simulink model "HopperRaibert"  (R2025a)
settings: Solver=VariableStepAuto  StartTime=0.0  StopTime=10.0  RelTol=1e-3
libraries: aru_toolbox x2, simulink x1
settings Model: Creator=Gavin  LastModifiedBy=Gavin
settings ExplorerConfigSet: InternalSimMechanicsExplorerSettings="<ExplorerConfiguration><canonicalview>default</canonicalview><TilePanel><TileInfo><Tiles Columns=\"1\" Count=\"1\" Height=\"832\" Rows=\"1\" Width=\"1462\"><Row Weight=\"1\"/><Column Weight=\"1\"/><Tile Height=\"1\" Width=\"1\" X=\"0\" Y=\"0\"/></Tiles></TileInfo><SceneInfo><SceneViewer><IsThisViewStd><IsStandardView>off</IsStandardView><StandardViewName>Front</StandardViewName></IsThisViewStd><BGColor><R>1</R><G>1</G><B>1</B><A>1</A></BGColor><Camera><DoPerspective>on</DoPerspective><Position><X>-0.15165999999999999</X><Y>3.9971199999999998</Y><Z>0.85099999999999998</Z></Position><Center><X>0</X><Y>0</Y><Z>0.10100000000000001</Z></Center><Up><X>0.0069873130929931429</X><Y>-0.18415619748295364</Y><Z>0.98287215464899591</Z></Up><XLim>1.8977346774231529</XLim><YLim>1.8977346774231529</YLim><ViewLimDist>0.01</ViewLimDist></Camera></SceneViewer></SceneInfo></TilePanel><MechEditorPanel><GfxPanelCameraMap><MapElement CameraMLId=\"Camera1\" GfxPanelIndex=\"0\"/></GfxPanelCameraMap><Cameras><Camera><Id>Camera1</Id><Value><Name>FollowBot</Name><NativeCamera><PositionTrackingFeature>Subsystem.Half_Baleka_Simscape_WIP.Planarising_Boom.Center_to_CameraUp.F</PositionTrackingFeature><CenterTrackingFeature>Subsystem.Half_Baleka_Simscape_WIP.Planarising_Boom.Center_to_Camera.B</CenterTrackingFeature><UpVectorTrackingFeature>Subsystem.Half_Baleka_Simscape_WIP.Planarising_Boom.Center_to_Camera.B</UpVectorTrackingFeature><CenterTrackingOrigin>on</CenterTrackingOrigin><UpVectorTrackingDirection>+Y</UpVectorTrackingDirection></NativeCamera></Value></Camera></Cameras><VideoCreator><IncludeTiles>All</IncludeTiles><IncludeTime>on</IncludeTime><IncludeWorldFrame>off</IncludeWorldFrame><PlaybackSpeedRatio>1</PlaybackSpeedRatio><FrameRate>30</FrameRate><FrameSize>auto</FrameSize><VideoFormat>MotionJPEGAVI</VideoFormat></VideoCreator></MechEditorPanel><PlaybackSettings><PlaybackSpeedFactor>1</PlaybackSpeedFactor></PlaybackSettings></ExplorerConfiguration>"

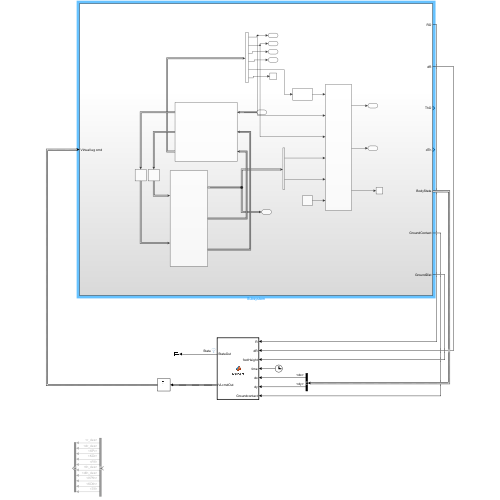
[thumbnail: Simulink's stored preview of the top-level diagram]
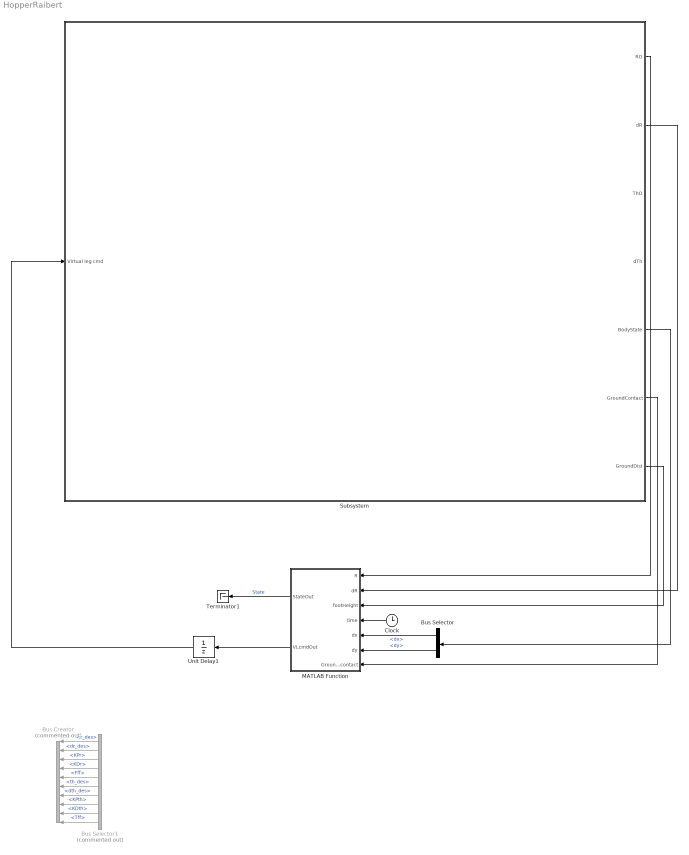
== system HopperRaibert ==
  Bus Creator : BusCreator  Commented=on  Inputs=10  OutDataTypeStr=Bus: VLcmd  NonVirtualBus=on
      settings: InheritFromInputs=off
  Bus Selector : BusSelector  OutputSignals=dx,dy
  Bus Selector1 : BusSelector  Commented=on  OutputSignals=r_des,dr_des,KPr,KDr,Fff,th_des,dth_des,KPth,KDth,Tff
  Clock : Clock
  MATLAB Function : MATLAB Function  TreatAsAtomicUnit=on
  Subsystem : Subsystem
  Terminator1 : Terminator
  Unit Delay1 : UnitDelay  SampleTime=-1  HasFrameUpgradeWarning=on
  wires:
  MATLAB Function/1(StateOut) -> Terminator1/1  "State"
  Subsystem/6(GroundContact) -> MATLAB Function/7(Groundcontact)
  Subsystem/2(dR) -> MATLAB Function/2(dR)
  Clock/1 -> MATLAB Function/4(time)
  Subsystem/1(RO) -> MATLAB Function/1(R)
  Subsystem/7(GroundDist) -> MATLAB Function/3(footHeight)
  Subsystem/5(BodyState) -> Bus Selector/1
  Bus Selector/1 -> MATLAB Function/5(dx)  "<dx>"
  Bus Selector/2 -> MATLAB Function/6(dy)  "<dy>"
  Bus Selector1/8 -> Bus Creator/8  "<KPth>"
  Bus Selector1/2 -> Bus Creator/2  "<dr_des>"
  Bus Selector1/4 -> Bus Creator/4  "<KDr>"
  Bus Selector1/7 -> Bus Creator/7  "<dth_des>"
  Bus Selector1/5 -> Bus Creator/5  "<Fff>"
  Bus Selector1/6 -> Bus Creator/6  "<th_des>"
  Bus Selector1/3 -> Bus Creator/3  "<KPr>"
  Bus Selector1/10 -> Bus Creator/10  "<Tff>"
  Bus Selector1/9 -> Bus Creator/9  "<KDth>"
  Bus Selector1/1 -> Bus Creator/1  "<r_des>"
  MATLAB Function/2(VLcmdOut) -> Unit Delay1/1
  Unit Delay1/1 -> Subsystem/1(Virtual leg cmd)

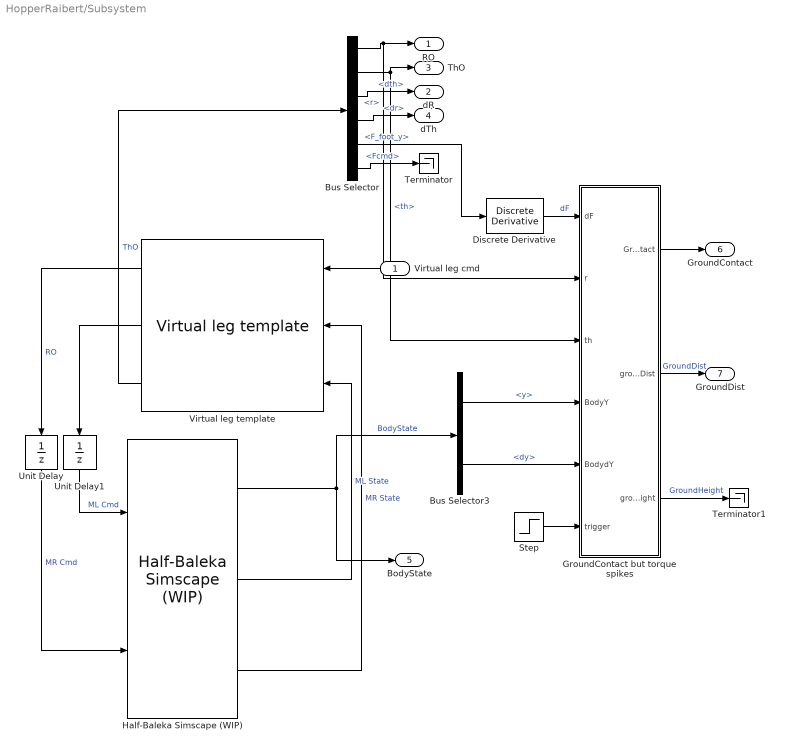
== system HopperRaibert/Subsystem ==
  Virtual leg cmd : Inport  OutDataTypeStr=Bus: VLcmd
  Bus Selector : BusSelector  OutputSignals=r,th,dth,dr,F_foot_y,Fcmd
  Bus Selector3 : BusSelector  OutputSignals=y,dy
  Discrete Derivative : simulink/Discrete/Discrete Derivative  gainval=1.0  ICPrevScaledInput=0.0  OutMin=[]  OutMax=[]  OutDataType=fixdt(1, 16)  OutScaling=2^-10  DoSatur=off
  GroundContact but torque spikes : MATLAB Function  TreatAsAtomicUnit=on
  Half-Baleka Simscape (WIP) : aru_toolbox/Baleka 2.5/Half-Baleka Simscape (WIP)  communication_rate=1000  GravityBool=on  mu_s=1  mu_k=0.9  foot_k=1e5  foot_d=1e4  y_start=0.8  dx_start=2  StartingMode=Zero (set Starting values manually)  LOffset=4.1  ROffset=-0.88  camX=4  camY=0.75
      settings: SourceProductName=ARU Toolbox
  Step : Step  Time=0.005  SampleTime=0
  Terminator : Terminator
  Terminator1 : Terminator
  Unit Delay : UnitDelay  SampleTime=-1  HasFrameUpgradeWarning=on
  Unit Delay1 : UnitDelay  SampleTime=-1  HasFrameUpgradeWarning=on
  Virtual leg template : aru_toolbox/Baleka 2.5/Virtual leg template  SystemSampleTime=-1  VariantActivationTime=update diagram  EmptyChoice=off  PassThrough=off  PassThroughVariantControl=(default)  EmptyChoiceVariantControl=(default)  AllowFlexibleInterface=on  Latency=0  AutoFrameSizeCalculation=off
      settings: SourceProductName=ARU Toolbox
  RO : Outport
  dR : Outport  Port=2
  ThO : Outport  Port=3
  dTh : Outport  Port=4
  BodyState : Outport  Port=5
  GroundContact : Outport  Port=6
  GroundDist : Outport  Port=7
  wires:
  Bus Selector/6 -> Terminator/1  "<Fcmd>"
  Bus Selector/4 -> dTh/1  "<dr>"
  Bus Selector/1 -> GroundContact but torque spikes/2(r), RO/1  "<r>"
  Unit Delay1/1 -> Half-Baleka Simscape (WIP)/1  "ML Cmd"
  Virtual leg cmd/1 -> Virtual leg template/1
  Virtual leg template/3 -> Bus Selector/1  "ThO"
  Half-Baleka Simscape (WIP)/3 -> Virtual leg template/2  "MR State"
  Half-Baleka Simscape (WIP)/2 -> Virtual leg template/3  "ML State"
  Virtual leg template/1 -> Unit Delay/1  "RO"
  Bus Selector/2 -> ThO/1, GroundContact but torque spikes/3(th)  "<th>"
  Unit Delay/1 -> Half-Baleka Simscape (WIP)/2  "MR Cmd"
  Half-Baleka Simscape (WIP)/1 -> BodyState/1, Bus Selector3/1  "BodyState"
  Bus Selector/5 -> Discrete Derivative/1  "<F_foot_y>"
  GroundContact but torque spikes/1(GroundContact) -> GroundContact/1
  Bus Selector/3 -> dR/1  "<dth>"
  Virtual leg template/2 -> Unit Delay1/1
  Bus Selector3/1 -> GroundContact but torque spikes/4(BodyY)  "<y>"
  Bus Selector3/2 -> GroundContact but torque spikes/5(BodydY)  "<dy>"
  GroundContact but torque spikes/3(groundHeight) -> Terminator1/1  "GroundHeight"
  Discrete Derivative/1 -> GroundContact but torque spikes/1(dF)  "dF"
  GroundContact but torque spikes/2(groundDist) -> GroundDist/1  "GroundDist"
  Step/1 -> GroundContact but torque spikes/6(trigger)

== matlab function HopperRaibert/MATLAB Function ==
  settings: updateMethod=DISCRETE  sampleTime=0.001
  data: R input; StateOut output; dR input; footHeight input; time input; dx input; dy input; VLcmdOut output Bus: VLcmd; Groundcontact input
function [StateOut, VLcmdOut]   = Raibert(R, dR,footHeight, time,dx, dy, Groundcontact)
    % Raibert hopping state machine
    persistent state landTime VLcmd x_f_des %dR
    % State variable
    % 0 = SETUP
    % 1 = FLIGHT
    % 2 = COMPRESSION
    % 3 = THRUST
    
    % Params:
    Ts = 0.15;
    Kdx = 0.1;
    dx_d = 2;


    x_f = dx*Ts/2 + Kdx*(dx - dx_d); % Foot placement
    % x_f = 0.1;
    
    if isempty(state)
        state = 0;
        x_f_des = 0;
        landTime = 99;
        % dR = 0;
        VLcmd.r_des = 0.45;
        VLcmd.dr_des =0;
        VLcmd.KPr = 1000;
        VLcmd.KDr =40;
        VLcmd.Fff =0;
        VLcmd.th_des = -pi/2 + asin(x_f/R);
        VLcmd.dth_des =0;
        VLcmd.KPth = 200;
        VLcmd.KDth = 20;
        VLcmd.Tff = 0;
        
    end

switch state
    case 0 % SETUP
        % Specific commands for first landing
        VLcmd.r_des = 0.45;
        VLcmd.dr_des =0;
        VLcmd.KPr = 1000;
        VLcmd.KDr =40;
        VLcmd.Fff =0;

        VLcmd.th_des = -pi/2 + asin(x_f/R);
        VLcmd.KPth = 200;
        VLcmd.KDth = 20;
        if Groundcontact % On foot touching ground go to COMPRESSION
            state = 2;
            landTime = time;
            x_f_des = x_f;

        end
    case 1 % FLIGHT
        % Brace for impact with high-ish spring
        VLcmd.r_des = 0.45;
        VLcmd.dr_des =0;
        VLcmd.KPr = 600;
        VLcmd.KDr =20;
        VLcmd.Fff = 0;
        % Position leg for landing
        VLcmd.th_des = -pi/2 +asin(x_f/R);
        VLcmd.dth_des = 0;
        VLcmd.KPth = 600;
        VLcmd.KDth = 20;

        if Groundcontact % On foot touching ground go to COMPRESSION
            state = 2;
            landTime = time;
        end
    case 2 % COMPRESSION
        % Let spring compress
        VLcmd.r_des = 0.45;
        VLcmd.dr_des =0;
        VLcmd.KPr = 900;
        VLcmd.KDr =10;
        VLcmd.Fff = 0;
        % Servo hip
        VLcmd.th_des = -pi/2- asin(x_f_des/R); 
        VLcmd.dth_des = 0;%(dx*R - dR*R*sin(th))/(cos(th)*R^2);
        VLcmd.KPth = 800;
        VLcmd.KDth = 50;
        % When leg stops compressing (dR = 0) go to THRUST
        if (((time-landTime)>0.05)&&(dR>0)) 
            state = 3;
        end
    case 3 % THRUST
        % Apply upwards thrust force
        VLcmd.r_des = 0.6;
        VLcmd.dr_des =0;
        VLcmd.KPr = 5000;
        VLcmd.KDr =0;
        VLcmd.Fff = 0;% 2000;

        % Servo hip
        VLcmd.th_des = -pi/2 - asin(x_f_des/R); 
        VLcmd.dth_des = 0;%(dx*R - dR*R*sin(th))/(cos(th)*R^2);
        VLcmd.KPth = 800;
        VLcmd.KDth = 50;

        if ~Groundcontact%&&(dy>0))% ||((th1>3*pi/2)||(th2<-pi/2))
            state =1;
        end

end
    VLcmdOut.r_des = VLcmd.r_des;
    VLcmdOut.dr_des = VLcmd.dr_des;
    VLcmdOut.KPr = VLcmd.KPr;
    VLcmdOut.KDr = VLcmd.KDr;
    VLcmdOut.Fff = VLcmd.Fff;

    VLcmdOut.th_des = VLcmd.th_des;
    VLcmdOut.dth_des = VLcmd.dth_des;
    VLcmdOut.KPth = VLcmd.KPth;
    VLcmdOut.KDth = VLcmd.KDth;
    VLcmdOut.Tff = VLcmd.Tff;

    StateOut = state;
end

== matlab function HopperRaibert/Subsystem/GroundContact but torque spikes ==
  settings: updateMethod=DISCRETE  sampleTime=0.001
  data: dF input; r input; th input; GroundContact output; BodyY input; groundDist output; groundHeight output; BodydY input; trigger input
function [GroundContact, groundDist, groundHeight]  = ImpactTorque(dF,r, th, BodyY, BodydY, trigger)
        % need to see how IRL torque spikes work, but we can do a veeery
        % rough guestimate here:
        persistent GroundContactpers;
        persistent GroundHeight;
        if isempty(GroundContactpers)
            GroundContactpers = false;
            GroundHeight = 0;
        end
        if trigger >0
        %     GroundContactpers = true;
        %     GroundHeight = BodyY  +sin(th)*r;
        % end

            if ~GroundContactpers % Impact sensing for gnd
               if (dF<-1.5e4) && (BodydY <0)
                GroundContactpers = true;
                GroundHeight = BodyY  +sin(th)*r; % - 0.004
               end
               groundDist=BodyY + sin(th)*r;
            else 
                % leg length calc for flight
                groundDist = BodyY + sin(th)*r;% - 0.004
                if BodydY >0
                    GroundContactpers = ~(groundDist>0.005+GroundHeight);
                end
            end

        else
            groundDist=BodyY + sin(th)*r;
        end
          
        GroundContact = GroundContactpers;
        groundHeight = GroundHeight;
end
